simulink model "PassiveModel"  (R2025b)
settings: Solver=FixedStepAuto  StartTime=0.0  StopTime=1.5  FixedStep=1e-6  MaxStep=1e-3  MinStep=1e-8  RelTol=1e-4
undefined symbols (not defined in the file or in its folder): cc, ks, kt, ms, mu
libraries: simulink x1
settings Model: SimulationMode=accelerator  Creator=khalid  LastModifiedBy=khalidwaleed
settings SolverCC: InitialStep=1e-5  ZeroCrossAlgorithm=Adaptive
settings DataIOCC: SaveTime=off
settings DebuggingCC: MaskedZcDiagnostic=none  IgnoredZcDiagnostic=none

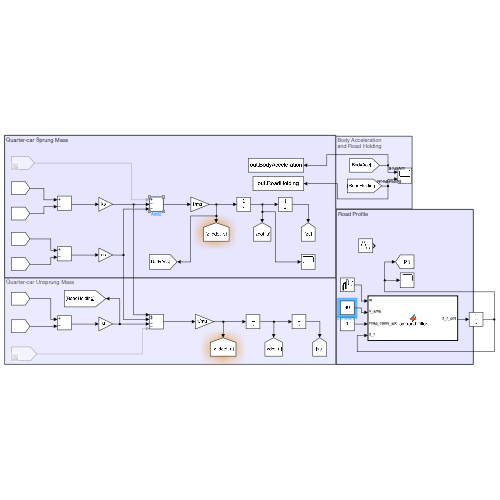
[thumbnail: Simulink's stored preview of the top-level diagram]
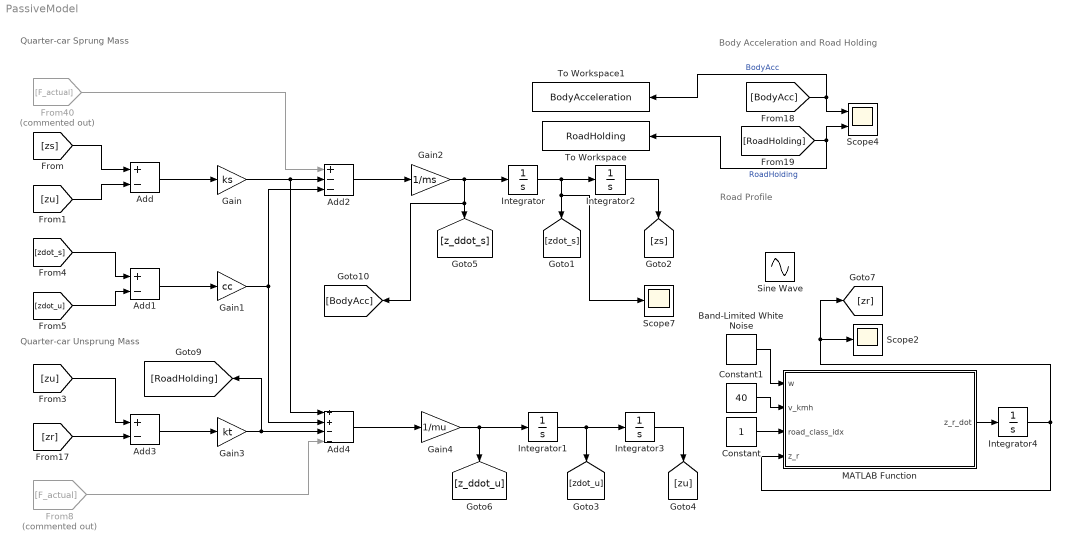
== system PassiveModel ==
  note: Road Profile
  note: Body Acceleration
      | and Road Holding
  note: Quarter-car Sprung Mass
  note: Quarter-car Unsprung Mass
  Add : Sum  Inputs=+-
  Add1 : Sum  Inputs=+-
  Add2 : Sum  Inputs=+--
  Add3 : Sum  Inputs=+-
  Add4 : Sum  Inputs=++--
  Band-Limited White Noise : simulink/Sources/Band-Limited White Noise  Cov=[1]  Ts=0.01  seed=[23341]
  Constant : Constant
  Constant1 : Constant  Value=40
  From40 : From  Commented=on  GotoTag=F_actual
  From8 : From  Commented=on  GotoTag=F_actual
  Gain : Gain  Gain=ks
  Gain1 : Gain  Gain=cc
  Gain2 : Gain  Gain=1/ms
  Gain3 : Gain  Gain=kt
  Gain4 : Gain  Gain=1/mu
  Integrator{,1..4} (5 alike) : Integrator
  MATLAB Function : MATLAB Function  TreatAsAtomicUnit=on
  Scope2 : Scope
      settings: ActiveDisplayYMinimum=-0.0076345988746295539  ActiveDisplayYMaximum=0.015995642543704076
  Scope4 : Scope  NumInputPorts=2
      settings: ActiveDisplayYMinimum=-1319.7407662714395  ActiveDisplayYMaximum=1443.7691557161784  DataLoggingVariableName=ScopeData5
  Scope7 : Scope
      settings: ActiveDisplayYMinimum=-0.076226191577344518  ActiveDisplayYMaximum=0.12589916007838611  DataLoggingVariableName=ScopeData7
  Sine Wave : Sin  Amplitude=0.03  Frequency=2*pi*1.3  SampleTime=0
  To Workspace : ToWorkspace  VariableName=RoadHolding  SaveFormat=Structure With Time  SampleTime=-1
  To Workspace1 : ToWorkspace  VariableName=BodyAcceleration  SaveFormat=Structure With Time  SampleTime=-1
  wires:
  [zdot_u] -> Add1/2
  Add3/1 -> Gain3/1
  Gain3/1 -> [RoadHolding], Add4/3
  [zs] -> Add/1
  Add1/1 -> Gain1/1
  [zr] -> Add3/2
  Add4/1 -> Gain4/1
  Integrator/1 -> Integrator2/1, [zdot_s], Scope7/1
  [zu] -> Add/2
  From8/1 -> Add4/4
  [zdot_s] -> Add1/1
  Gain2/1 -> Integrator/1, [BodyAcc], [z_ddot_s]
  Gain/1 -> Add4/1, Add2/2
  Add/1 -> Gain/1
  Gain4/1 -> Integrator1/1, [z_ddot_u]
  [zu] -> Add3/1
  Add2/1 -> Gain2/1
  Integrator3/1 -> [zu]
  Integrator1/1 -> Integrator3/1, [zdot_u]
  Integrator2/1 -> [zs]
  From40/1 -> Add2/1
  [BodyAcc] -> Scope4/1, To Workspace1/1  "BodyAcc"
  [RoadHolding] -> Scope4/2, To Workspace/1  "RoadHolding"
  Gain1/1 -> Add4/2, Add2/3
  Band-Limited White Noise/1 -> MATLAB Function/1(w)
  MATLAB Function/1(z_r_dot) -> Integrator4/1
  Integrator4/1 -> Scope2/1, [zr], MATLAB Function/4(z_r)
  Constant/1 -> MATLAB Function/3(road_class_idx)
  Constant1/1 -> MATLAB Function/2(v_kmh)

== matlab function PassiveModel/MATLAB Function ==
  data: w input; z_r_dot output; v_kmh input; road_class_idx input; z_r input
function z_r_dot = iso_road_filter(w, v_kmh, road_class_idx, z_r)
    % Inputs:
    %   w              - White noise input signal
    %   v_kmh          - Vehicle speed in km/h from workspace
    %   road_class_idx - 1 for Class B, 2 for Class D
    %   z_r            - Current road displacement (feedback loop)
    
    % Constants
    n_0 = 0.1;   % Reference spatial frequency (cycles/m)
    n_c = 0.01;  % Low frequency cut-off (cycles/m)
    
    % Convert speed from km/h to m/s
    v = v_kmh / 3.6; 
    
    % Select roughness coefficient based on road class index
    if road_class_idx == 1
        G_0 = 64e-6;   % Class B nominal
    else
        G_0 = 1024e-6; % Class D nominal
    end
    
    % Avoid division by zero if vehicle stops
    if v < 0.1
        v = 0.1;
    end
    
    % Compute the derivative of the road profile displacement
    z_r_dot = -2*pi*n_c*v*z_r + 2*pi*n_0*sqrt(G_0*v)*w;
end
